simulink model "advanced_robotics_control"  (R2024a)
settings: Solver=ode1  StartTime=0.0  StopTime=5  FixedStep=0.01  RelTol=1e-3
settings Model: Creator=gujun  LastModifiedBy=jun
settings RTWCC: GPUComputeCapability=3.5

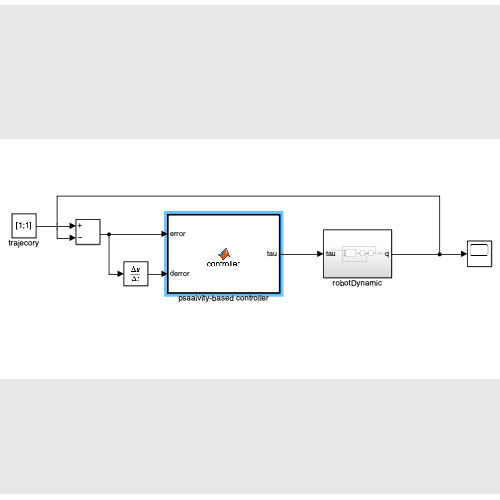
[thumbnail: Simulink's stored preview of the top-level diagram]
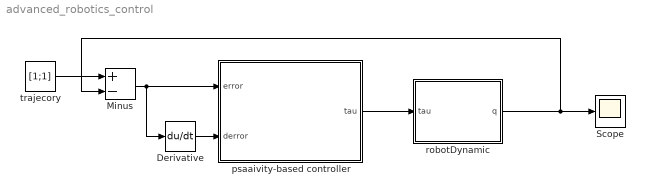
== system advanced_robotics_control ==
  Derivative : Derivative
  Minus : Sum  Inputs=+-
  Scope : Scope
  psaaivity-based controller : MATLAB Function  TreatAsAtomicUnit=on
  robotDynamic : Subsystem
  trajecory : Constant  Value=[1;1]
  wires:
  trajecory/1 -> Minus/1
  Minus/1 -> Derivative/1, psaaivity-based controller/1(error)
  Derivative/1 -> psaaivity-based controller/2(derror)
  psaaivity-based controller/1(tau) -> robotDynamic/1(tau)
  robotDynamic/1(q) -> Scope/1, Minus/2

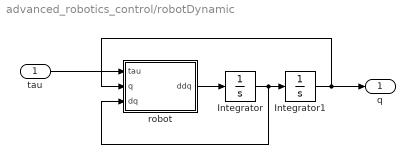
== system advanced_robotics_control/robotDynamic ==
  tau : Inport
  Integrator : Integrator
  Integrator1 : Integrator
  robot : MATLAB Function  TreatAsAtomicUnit=on
  q : Outport
  wires:
  robot/1(ddq) -> Integrator/1
  tau/1 -> robot/1(tau)
  Integrator1/1 -> q/1, robot/2(q)
  Integrator/1 -> Integrator1/1, robot/3(dq)

== matlab function advanced_robotics_control/psaaivity-based controller ==
  data: error input; tau output; derror input
function tau = controller(error, derror)

kp = [10, 0;
       0, 4];


kd = [1, 0;
        0, 0.3];

tau = kp * error + kd * derror;

== matlab function advanced_robotics_control/robotDynamic/robot ==
  data: tau input size=2; ddq output size=2; q input size=2; dq input size=2
function ddq = robot(tau, q, dq)

I1 = 0.05;
m1 = 1.5;
lg1 = 0.2;

I2 = 0.01;
m2 = 0.5;
lg2 = 0.2;

g = 9.8;
% g = 0;

a1 = I1 + I2 + m2 * lg1 * lg1;
a2 = m2 * lg1 * lg2;
a3 = I2 ;

L = [lg1, 0;
        0, lg2];

M = L * [a1 + 2 * a2 * cos(q(2)), a3 - a2 * cos(q(2));
        a3 + a2 * cos(q(2)), a3 / lg2];

h = L * [-a2 * sin(q(2)) * (2 * dq(1) * dq(2) + dq(2) * dq(2)) - (m1 + m2) * lg1 * g * sin(q(1)) - m2 * lg2 * g * sin(q(1) + q(2));
        -a2 * sin(q(2)) * dq(1) * dq(2) - m2 * lg2 * g * sin(q(1) + q(2))];

ddq = M \ (tau - h);
